simulink model "AOO_3K04"  (R2022a)
settings: Solver=FixedStepAuto  StartTime=0.0  StopTime=10.0  FixedStep=1e-3  RelTol=1e-3  EnableMultiTasking=on
undefined symbols (not defined in the file): D10, D11, D2, D4, D5, D8, D9, PTA0, PTA2, PTB23, PTB9, PTC4, PTD0, PTD2
libraries: frdmk64flib x7
settings Model: ExtModeTrigDuration=5  Creator=patri  LastModifiedBy=patri
settings OptimizationCC: EnhancedBackFolding=on  PassReuseOutputArgsAs=Individual arguments  ZeroExternalMemoryAtStartup=off  ZeroInternalMemoryAtStartup=off  MaxStackSize=64  OptimizeBlockOrder=speed  DifferentSizesBufferReuse=on  OptimizationCustomize=off  EfficientTunableParamExpr=on
settings DebuggingCC: ParameterTunabilityLossMsg=error
settings HardwareCC: ProdBitPerPointer=32  ProdBitPerSizeT=32  ProdBitPerPtrDiffT=32  ProdLargestAtomicInteger=Long  ProdLargestAtomicFloat=Double  ProdWordSize=32  ProdHWDeviceType=ARM Compatible->ARM Cortex
settings SFSimCC: MATLABDynamicMemAlloc=off
settings RTWCC: SystemTargetFile=ert.tlc  HardwareBoard=NXP FRDM-K64F  TLCOptions="-aInlineSetEventsForThisBaseRateFcn=TLC_FALSE -aSuppressMultiTaskScheduler=TLC_FALSE  -aRateBasedStepFcn=0"  TemplateMakefile=ert_default_tmf  Toolchain=GNU Tools for ARM Embedded Processors
settings CodeAppCC: ForceParamTrailComments=on  IgnoreCustomStorageClasses=off  OperatorAnnotations=on  SimulinkDataObjDesc=on  SFDataObjDesc=on  InsertBlockDesc=on
settings ERTTargetCC: ExtModeTransport=4  ExtModeMexFile=sendToCommService

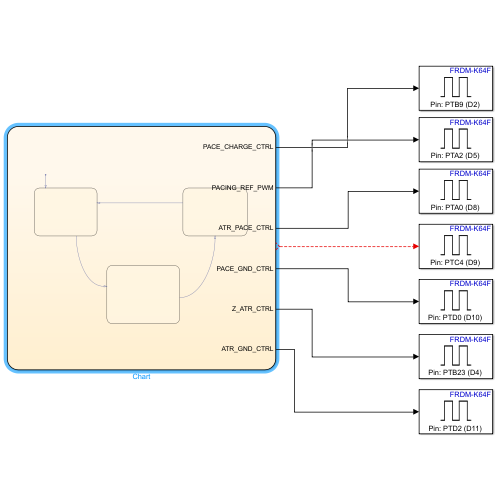
[thumbnail: Simulink's stored preview of the top-level diagram]
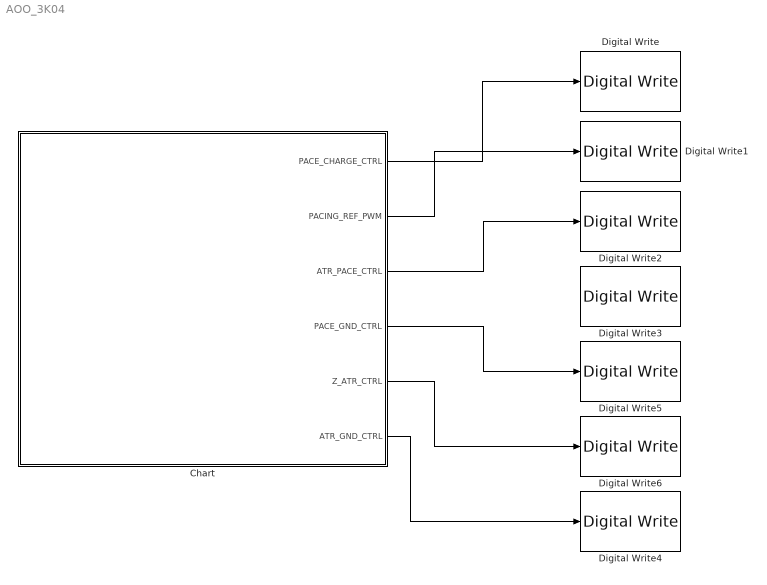
== system AOO_3K04 ==
  Chart : Stateflow chart  TreatAsAtomicUnit=on
  Digital Write : frdmk64flib/Digital Write  Whichpin=PTB9 (D2)
  Digital Write1 : frdmk64flib/Digital Write  Whichpin=PTA2 (D5)
  Digital Write2 : frdmk64flib/Digital Write  Whichpin=PTA0 (D8)
  Digital Write3 : frdmk64flib/Digital Write  Whichpin=PTC4 (D9)
  Digital Write4 : frdmk64flib/Digital Write  Whichpin=PTD2 (D11)
  Digital Write5 : frdmk64flib/Digital Write  Whichpin=PTD0 (D10)
  Digital Write6 : frdmk64flib/Digital Write  Whichpin=PTB23 (D4)
  wires:
  Chart/1(PACE_CHARGE_CTRL) -> Digital Write/1
  Chart/2(PACING_REF_PWM) -> Digital Write1/1
  Chart/3(ATR_PACE_CTRL) -> Digital Write2/1
  ? -> Digital Write3/1
  Chart/4(PACE_GND_CTRL) -> Digital Write5/1
  Chart/5(Z_ATR_CTRL) -> Digital Write6/1
  Chart/6(ATR_GND_CTRL) -> Digital Write4/1

== stateflow chart AOO_3K04/Chart ==
  state Charging_C22
    entry:
    ATR_PACE_CTRL = false;
    PACING_REF_PWM = 2000;
    PACE_CHARGE_CTRL = true;
  state Discharging_C22
    entry:
    PACE_GND_CTRL = true;
    ATR_PACE_CTRL = false;
    Z_ATR_CTRL = false;
    ATR_GND_CTRL = true;
  state ATR_Pacing
    entry:
    PACE_CHARGE_CTRL = false;
    PACE_GND_CTRL = true;
    ATR_PACE_CTRL = true;
    ATR_GND_CTRL = false;
    Z_ATR_CTRL = false;
  (default) -> Charging_C22
  Discharging_C22 -> Charging_C22 : after(1000,msec)
  ATR_Pacing -> Discharging_C22 : after(1000,msec)
  Charging_C22 -> ATR_Pacing : after(1000,msec)
  data: PACE_CHARGE_CTRL output; PACING_REF_PWM output; ATR_PACE_CTRL output; PACE_GND_CTRL output; Z_ATR_CTRL output; ATR_GND_CTRL output
